simulink model "Guidance"  (R2023a)
settings: Solver=ode1  StartTime=0.0  StopTime=inf  FixedStep=0.005  RelTol=1e-3  EnableMultiTasking=on
libraries: etargetslib x2, arduinolib x2, svdutilitieslib x1
settings Model: ExtModeTrigDuration=2  Creator=Ali  LastModifiedBy=Ali
settings OptimizationCC: EnhancedBackFolding=on  PassReuseOutputArgsAs=Individual arguments  ZeroExternalMemoryAtStartup=off  ZeroInternalMemoryAtStartup=off  MaxStackSize=64  OptimizeBlockOrder=speed  DifferentSizesBufferReuse=on  OptimizationCustomize=off  EfficientTunableParamExpr=on
settings DebuggingCC: ParameterTunabilityLossMsg=error
settings HardwareCC: ProdBitPerPointer=32  ProdBitPerSizeT=32  ProdBitPerPtrDiffT=32  ProdLargestAtomicInteger=Long  ProdLargestAtomicFloat=Double  ProdWordSize=32  ProdHWDeviceType=ARM Compatible->ARM Cortex
settings SFSimCC: MATLABDynamicMemAlloc=off
settings RTWCC: Description=Embedded Coder  SystemTargetFile=ert.tlc  HardwareBoard=Arduino Due  TemplateMakefile=ert_default_tmf  Toolchain=Arduino ARM  BuildConfiguration=Faster Runs
settings CodeAppCC: ForceParamTrailComments=on  IgnoreCustomStorageClasses=off  OperatorAnnotations=on  SimulinkDataObjDesc=on  SFDataObjDesc=on  InsertBlockDesc=on
settings ERTTargetCC: SupportContinuousTime=on  SupportVariableSizeSignals=on  ExtModeTransport=3  ExtModeStaticAlloc=on  ExtModeAutomaticAllocSize=off  ExtModeStaticAllocSize=24576  ExtModeMexFile=ext_xcp  ExtModeIntrfLevel=Level2 - Open

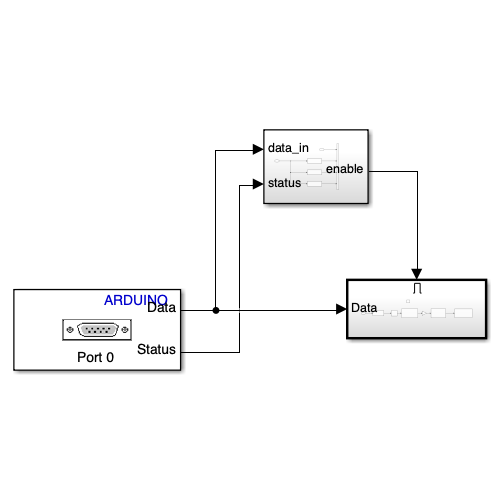
[thumbnail: Simulink's stored preview of the top-level diagram]
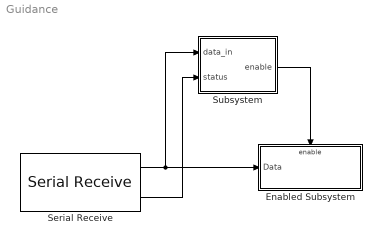
== system Guidance ==
  Enabled Subsystem : Subsystem  TreatAsAtomicUnit=on
  Serial Receive : arduinolib/Serial Receive  isARMArch=on  portNumber=0  DataType=uint8  Datalength=32  SampleTime=0.005  showOutStatus=on  blockPlatform=arduino
  Subsystem : Subsystem
  wires:
  Serial Receive/1 -> Subsystem/1(data_in), Enabled Subsystem/1(Data)
  Serial Receive/2 -> Subsystem/2(status)
  Subsystem/1(enable) -> Enabled Subsystem/Enable

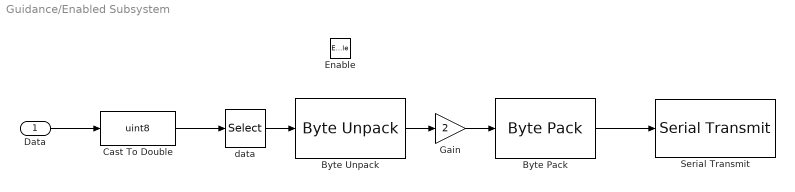
== system Guidance/Enabled Subsystem ==
  Data : Inport
  Enable : EnablePort
  Byte Pack : svdutilitieslib/Byte Pack  maskPackedDataType=uint8  datatypes={'single'}  byteAlign=1  blockPlatform=arduinoert
  Byte Unpack : etargetslib/Byte Unpack  dimensions={[6]}  datatypes={'single'}  byteAlign=1
      settings: LibrarySourceBlock=embeddedtargetslib/Host Communication/Byte Unpack
  Cast To Double : DataTypeConversion  OutDataTypeStr=uint8  SaturateOnIntegerOverflow=off  RndMeth=Floor
  Gain : Gain  Gain=2
  Serial Transmit : arduinolib/Serial Transmit  portNumber=0  sendmode=write  sendformat=Decimal  floatprecision=2  blockPlatform=arduino
  data : Selector  InputPortWidth=32  IndexOptions=Index vector (dialog)  Indices=[3:26]  OutputSizes=1
  wires:
  Byte Pack/1 -> Serial Transmit/1
  Cast To Double/1 -> data/1
  Data/1 -> Cast To Double/1
  data/1 -> Byte Unpack/1
  Byte Unpack/1 -> Gain/1
  Gain/1 -> Byte Pack/1

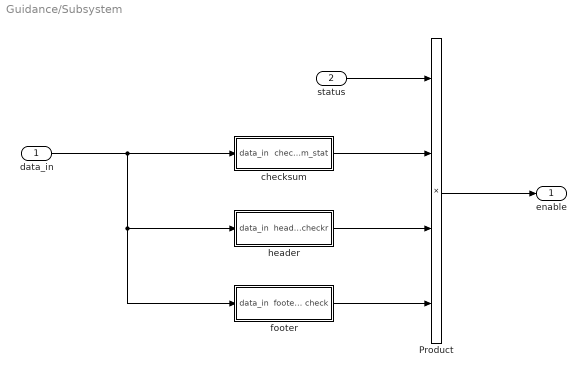
== system Guidance/Subsystem ==
  data_in : Inport
  status : Inport  Port=2
  Product : Product  Inputs=4
  checksum : Subsystem
  footer : Subsystem
  header : Subsystem
  enable : Outport
  wires:
  Product/1 -> enable/1
  status/1 -> Product/1
  data_in/1 -> footer/1(data_in), header/1(data_in), checksum/1(data_in)
  checksum/1(checksum_stat) -> Product/2
  header/1(heade_checkr) -> Product/3
  footer/1(footer check) -> Product/4

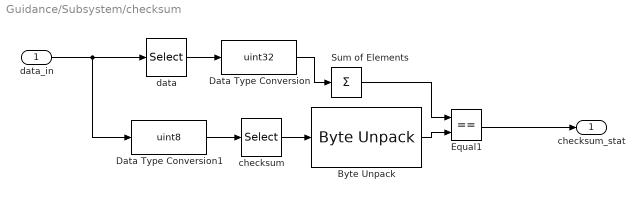
== system Guidance/Subsystem/checksum ==
  data_in : Inport
  Byte Unpack : etargetslib/Byte Unpack  dimensions={[1]}  datatypes={'uint32'}  byteAlign=1
      settings: LibrarySourceBlock=embeddedtargetslib/Host Communication/Byte Unpack
  Data Type Conversion : DataTypeConversion  OutDataTypeStr=uint32  SaturateOnIntegerOverflow=off  RndMeth=Floor
  Data Type Conversion1 : DataTypeConversion  OutDataTypeStr=uint8  SaturateOnIntegerOverflow=off  RndMeth=Floor
  Equal1 : RelationalOperator  Operator===  OutDataTypeStr=boolean  RndMeth=Simplest  InputSameDT=off
  Sum of Elements : Sum  Inputs=+
  checksum : Selector  InputPortWidth=32  IndexOptions=Index vector (dialog)  Indices=[27:30]  OutputSizes=1
  data : Selector  InputPortWidth=32  IndexOptions=Index vector (dialog)  Indices=[3:26]  OutputSizes=1
  checksum_stat : Outport
  wires:
  Sum of Elements/1 -> Equal1/1
  data_in/1 -> Data Type Conversion1/1, data/1
  Byte Unpack/1 -> Equal1/2
  Data Type Conversion1/1 -> checksum/1
  Equal1/1 -> checksum_stat/1
  data/1 -> Data Type Conversion/1
  checksum/1 -> Byte Unpack/1
  Data Type Conversion/1 -> Sum of Elements/1

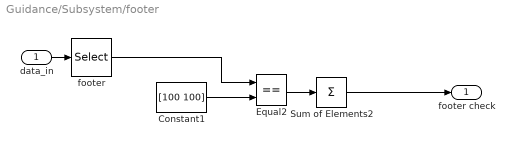
== system Guidance/Subsystem/footer ==
  data_in : Inport
  Constant1 : Constant  Value=[100 100]
  Equal2 : RelationalOperator  Operator===  OutDataTypeStr=boolean  RndMeth=Simplest  InputSameDT=off
  Sum of Elements2 : Sum  Inputs=+
  footer : Selector  InputPortWidth=32  IndexOptions=Index vector (dialog)  Indices=[31 32]  OutputSizes=1
  footer check : Outport
  wires:
  Sum of Elements2/1 -> footer check/1
  data_in/1 -> footer/1
  Constant1/1 -> Equal2/2
  footer/1 -> Equal2/1
  Equal2/1 -> Sum of Elements2/1

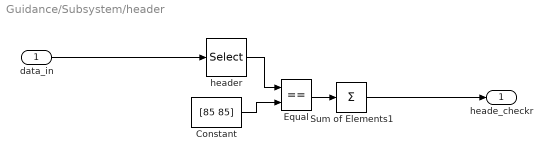
== system Guidance/Subsystem/header ==
  data_in : Inport
  Constant : Constant  Value=[85 85]
  Equal : RelationalOperator  Operator===  OutDataTypeStr=boolean  RndMeth=Simplest  InputSameDT=off
  Sum of Elements1 : Sum  Inputs=+
  header : Selector  InputPortWidth=32  IndexOptions=Index vector (dialog)  Indices=[1 2]  OutputSizes=1
  heade_checkr : Outport
  wires:
  data_in/1 -> header/1
  Sum of Elements1/1 -> heade_checkr/1
  Constant/1 -> Equal/2
  header/1 -> Equal/1
  Equal/1 -> Sum of Elements1/1
